simulink model "ControlArduinoLazoCerrado"  (R2015a)
settings: Solver=ode45  StartTime=0.0  StopTime=15  RelTol=1e-3
undefined symbols (not defined in the file or in its folder): serial
libraries: instrumentlib x3
settings Model: Creator=DS  LastModifiedBy=eduar
settings DebuggingCC: UnderspecifiedInitializationDetection=Classic  MergeDetectMultiDrivingBlocksExec=none  SolverPrmCheckMsg=warning  FcnCallInpInsideContextMsg=EnableAllAsWarning  StateNameClashWarn=warning

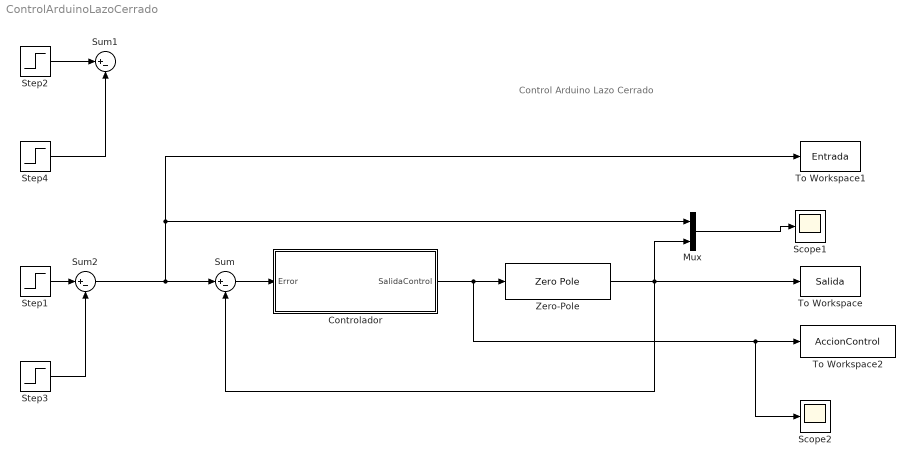
== system ControlArduinoLazoCerrado ==
  note: Control Arduino Lazo Cerrado
  Controlador : Subsystem
  Mux : Mux  Inputs=2
  Scope1 : Scope
      settings: TimeRange=6  YMin=165  YMax=200
  Scope2 : Scope
      settings: TimeRange=6  YMin=98.25  YMax=102.5
  Step1 : Step  After=200  SampleTime=0
  Step2 : Step  After=100  SampleTime=0
  Step3 : Step  Time=5  After=80  SampleTime=0
  Step4 : Step  Time=5  After=50  SampleTime=0
  Sum : Sum  Inputs=|+-
  Sum1 : Sum  Inputs=|+-
  Sum2 : Sum  Inputs=|+-
  To Workspace : ToWorkspace  VariableName=Salida  SampleTime=-1
      settings: Save2DSignal=2-D array (concatenate along first dimension)
  To Workspace1 : ToWorkspace  VariableName=Entrada  SaveFormat=Structure With Time  SampleTime=-1
  To Workspace2 : ToWorkspace  VariableName=AccionControl  SaveFormat=Structure With Time  SampleTime=-1
      settings: Save2DSignal=2-D array (concatenate along first dimension)
  Zero-Pole : ZeroPole  Zeros=[]  Poles=[-3 -5 -4]  Gain=[100]
  wires:
  Mux/1 -> Scope1/1
  Sum/1 -> Controlador/1(Error)
  Zero-Pole/1 -> To Workspace/1, Sum/2, Mux/2
  Controlador/1(SalidaControl) -> Scope2/1, To Workspace2/1, Zero-Pole/1
  Step2/1 -> Sum1/1
  Step4/1 -> Sum1/2
  Step1/1 -> Sum2/1
  Step3/1 -> Sum2/2
  Sum2/1 -> To Workspace1/1, Mux/1, Sum/1

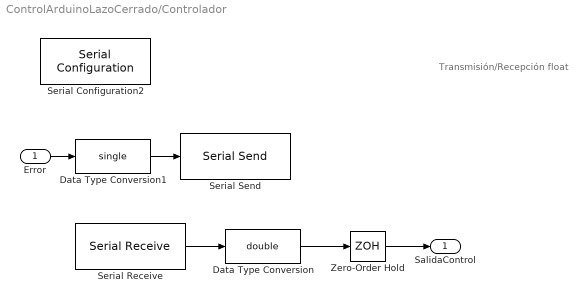
== system ControlArduinoLazoCerrado/Controlador ==
  note: Transmisión/Recepción float
  Error : Inport
  Data Type Conversion : DataTypeConversion  OutDataTypeStr=double  SampleTime=0.01
  Data Type Conversion1 : DataTypeConversion  OutDataTypeStr=single  SampleTime=0.01
  Serial Configuration2 : instrumentlib/Serial Configuration  Priority=-200000  ComPortMenu=COM4  ComPort=COM4  ObjConstructor=serial('COM4');  BaudRate=115200  DataBits=8  Parity=none  StopBits=1  FlowControl=none  Timeout=10  ByteOrder=LittleEndian
  Serial Receive : instrumentlib/Serial Receive  ComPortMenu=COM4  ComPort=COM4  ObjConstructor=serial('COM4');  Terminator=<none>  DataSize=[1 1]  DataType=single  EnableBlockingMode=on  ActionDataUnavailable=Output last received value  CustomValue=0  SampleTime=0.01
  Serial Send : instrumentlib/Serial Send  ComPortMenu=COM4  ComPort=COM4  ObjConstructor=serial('COM4');  Terminator=<none>  EnableBlockingMode=on
  Zero-Order Hold : ZeroOrderHold  SampleTime=0.01
  SalidaControl : Outport
  wires:
  Data Type Conversion/1 -> Zero-Order Hold/1
  Error/1 -> Data Type Conversion1/1
  Zero-Order Hold/1 -> SalidaControl/1
  Serial Receive/1 -> Data Type Conversion/1
  Data Type Conversion1/1 -> Serial Send/1
